simulink model "CLA_Sample"  (R2022b)
settings: Solver=FixedStepAuto  StartTime=0.0  StopTime=Inf  RelTol=1e-3  EnableMultiTasking=on
model workspace (MAT data in the model file):
  ADC_Gain = 1241.21212121
  DAC_Gain = 0.000805860805861
  Inductor_Current_Divider_Gain_Phase_A = 33.4
  Inductor_Current_Divider_Gain_Phase_B = 33.4
  Vbulk_Divider_Gain = 276.854928018
  Vin_Divider_Gain = 556.17352614
undefined symbols (not defined in the file or in its folder): GPTRIP1SEL, GPTRIP2SEL, SCI_A_Transmit, SCI_A_Transmit_Current_Suffix, SCI_A_Transmit_one_shot_Suffix, SCI_A_Transmit_Polarity_Suffix, SCI_A_Transmit_relay_Suffix, SCI_A_Transmit_Vbulk_Suffix, SCI_A_Transmit_Vin_rms_Suffix, SCI_A_Transmit_Vin_Suffix, SCI_A_Transmit_Vmid_Suffix, SCI_A_Transmit_Vp_Suffix, SCI_A_Transmit_Vpfc_Suffix, TZ1, TZ2
libraries: c280xlib x33, simulink x17, c2802xlib x15, c2000lib x1, c2806xlib x1
(part 1 of 5)
settings Model: ExtModeTrigDuration=8  Creator=natchammaimuthu  LastModifiedBy=hlaingwin
settings OptimizationCC: DefaultUnderspecifiedDataType=single  EnhancedBackFolding=on  PassReuseOutputArgsAs=Individual arguments  MaxStackSize=1024  OptimizeBlockOrder=speed  DifferentSizesBufferReuse=on  OptimizationCustomize=off  DenormalBehavior=FlushToZero  EfficientTunableParamExpr=on
settings DebuggingCC: MultiTaskDSMMsg=none  ParameterPrecisionLossMsg=none  ParameterTunabilityLossMsg=error
settings HardwareCC: ProdBitPerChar=16  ProdBitPerInt=16  ProdBitPerPointer=32  ProdBitPerSizeT=32  ProdBitPerPtrDiffT=32  ProdLargestAtomicInteger=Integer  ProdLargestAtomicFloat=None  ProdWordSize=16  ProdLongLongMode=on  ProdHWDeviceType=Texas Instruments->C2000
settings SFSimCC: MATLABDynamicMemAlloc=off
settings RTWCC: Description=Embedded Coder  SystemTargetFile=ert.tlc  HardwareBoard=TI Piccolo F2806x  TLCOptions=-aInlineSetEventsForThisBaseRateFcn=TLC_FALSE -aSuppressMultiTaskScheduler=TLC_FALSE -aRateBasedStepFcn=1  TemplateMakefile=ert_default_tmf  Toolchain=Texas Instruments Code Composer Studio (C2000)
settings CodeAppCC: ForceParamTrailComments=on  IgnoreCustomStorageClasses=off  OperatorAnnotations=on  SimulinkDataObjDesc=on  SFDataObjDesc=on  InsertBlockDesc=on
settings ERTTargetCC: CodeReplacementLibrary=TI C28x  ExtModeTransport=4  ExtModeStaticAlloc=on  ExtModeAutomaticAllocSize=off  ExtModeMexFile=ext_xcp  ExtModeIntrfLevel=Level2 - Open

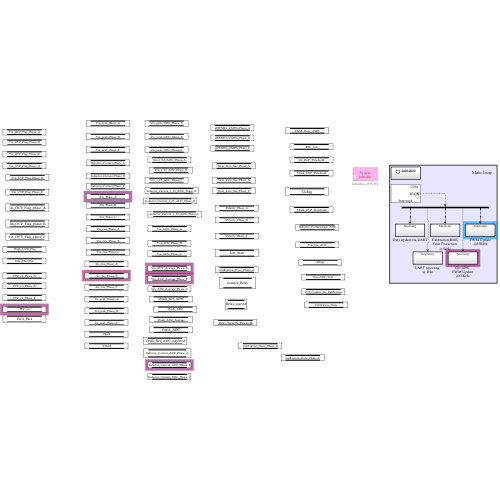
[thumbnail: Simulink's stored preview of the top-level diagram]
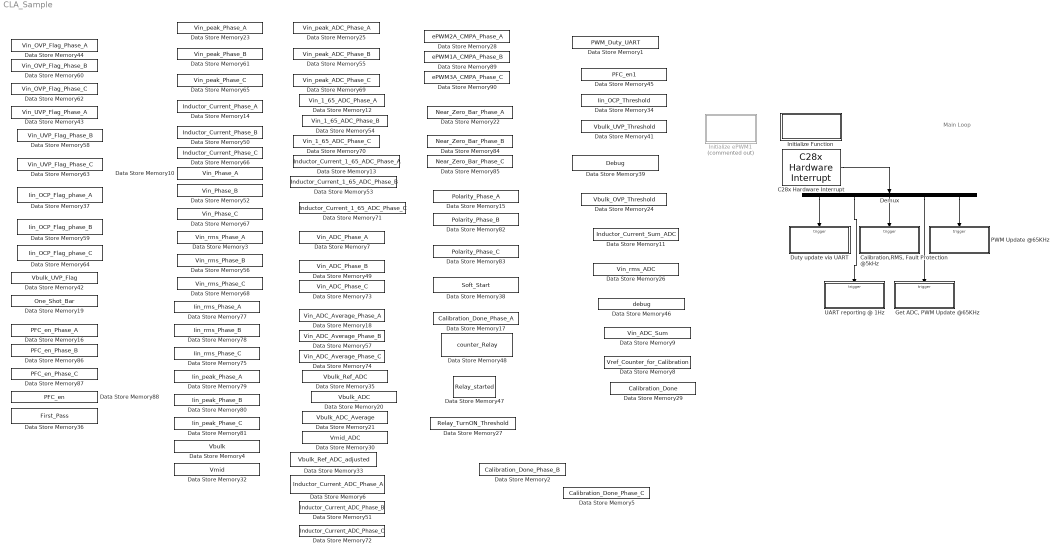
== system CLA_Sample ==
  note: Main Loop
  C28x Hardware Interrupt : c2000lib/Scheduling/C28x Hardware Interrupt  irqnumbers=[9 3 3 3 1]  pienumbers=[1 7 4 1 1]  irqpriorities=[10 9 8 7 6]  irqpreempts=[1 1 1 0 0]  showinput=off  dspchiptype=C280X
  "Calibration,RMS, Fault Protection @5kHz" : Subsystem  TreatAsAtomicUnit=on
  Data Store Memory1 : DataStoreMemory  DataStoreName=PWM_Duty_UART  WriteAfterWriteMsg=warning  InitialValue=5  ShowAdditionalParam=off  OutDataTypeStr=double
  Data Store Memory10 : DataStoreMemory  DataStoreName=Vin_Phase_A  WriteAfterWriteMsg=warning  ShowAdditionalParam=off  OutDataTypeStr=double
  Data Store Memory11 : DataStoreMemory  DataStoreName=Inductor_Current_Sum_ADC  WriteAfterWriteMsg=warning  ShowAdditionalParam=off  OutDataTypeStr=double
  Data Store Memory12 : DataStoreMemory  DataStoreName=Vin_1_65_ADC_Phase_A  WriteAfterWriteMsg=warning  ShowAdditionalParam=off  OutDataTypeStr=double
  Data Store Memory13 : DataStoreMemory  DataStoreName=Inductor_Current_1_65_ADC_Phase_A  WriteAfterWriteMsg=warning  ShowAdditionalParam=off  OutDataTypeStr=double
  Data Store Memory14 : DataStoreMemory  DataStoreName=Inductor_Current_Phase_A  WriteAfterWriteMsg=warning  ShowAdditionalParam=off  OutDataTypeStr=double
  Data Store Memory15 : DataStoreMemory  DataStoreName=Polarity_Phase_A  WriteAfterWriteMsg=warning  InitialValue=10  ShowAdditionalParam=off
  Data Store Memory16 : DataStoreMemory  DataStoreName=PFC_en_Phase_A  WriteAfterWriteMsg=warning  ShowAdditionalParam=off
  Data Store Memory17 : DataStoreMemory  DataStoreName=Calibration_Done_Phase_A  WriteAfterWriteMsg=warning  ShowAdditionalParam=off  OutDataTypeStr=double
  Data Store Memory18 : DataStoreMemory  DataStoreName=Vin_ADC_Average_Phase_A  WriteAfterWriteMsg=warning  ShowAdditionalParam=off
  Data Store Memory19 : DataStoreMemory  DataStoreName=One_Shot_Bar  WriteAfterWriteMsg=warning  InitialValue=1  ShowAdditionalParam=off  OutDataTypeStr=double
  Data Store Memory2 : DataStoreMemory  DataStoreName=Calibration_Done_Phase_B  WriteAfterWriteMsg=warning  ShowAdditionalParam=off  OutDataTypeStr=double
  Data Store Memory20 : DataStoreMemory  DataStoreName=Vbulk_ADC  WriteAfterWriteMsg=warning  ShowAdditionalParam=off
  Data Store Memory21 : DataStoreMemory  DataStoreName=Vbulk_ADC_Average  WriteAfterWriteMsg=warning  ShowAdditionalParam=off
  Data Store Memory22 : DataStoreMemory  DataStoreName=Near_Zero_Bar_Phase_A  WriteAfterWriteMsg=warning  InitialValue=10  ShowAdditionalParam=off
  Data Store Memory23 : DataStoreMemory  DataStoreName=Vin_peak_Phase_A  WriteAfterWriteMsg=warning  ShowAdditionalParam=off  OutDataTypeStr=double
  Data Store Memory24 : DataStoreMemory  DataStoreName=Vbulk_OVP_Threshold  WriteAfterWriteMsg=warning  InitialValue=100  ShowAdditionalParam=off
  Data Store Memory25 : DataStoreMemory  DataStoreName=Vin_peak_ADC_Phase_A  WriteAfterWriteMsg=warning  ShowAdditionalParam=off  OutDataTypeStr=double
  Data Store Memory26 : DataStoreMemory  DataStoreName=Vin_rms_ADC  WriteAfterWriteMsg=warning  InitialValue=10  ShowAdditionalParam=off
  Data Store Memory27 : DataStoreMemory  DataStoreName=Relay_TurnON_Threshold  WriteAfterWriteMsg=warning  InitialValue=10  ShowAdditionalParam=off
  Data Store Memory28 : DataStoreMemory  DataStoreName=ePWM2A_CMPA_Phase_A  WriteAfterWriteMsg=warning  ShowAdditionalParam=off
  Data Store Memory29 : DataStoreMemory  DataStoreName=Calibration_Done  WriteAfterWriteMsg=warning  ShowAdditionalParam=off  OutDataTypeStr=double
  Data Store Memory3 : DataStoreMemory  DataStoreName=Vin_rms_Phase_A  WriteAfterWriteMsg=warning  InitialValue=10  ShowAdditionalParam=off
  Data Store Memory30 : DataStoreMemory  DataStoreName=Vmid_ADC  WriteAfterWriteMsg=warning  InitialValue=10  ShowAdditionalParam=off  OutDataTypeStr=double
  Data Store Memory32 : DataStoreMemory  DataStoreName=Vmid  WriteAfterWriteMsg=warning  InitialValue=10  ShowAdditionalParam=off  OutDataTypeStr=double
  Data Store Memory33 : DataStoreMemory  DataStoreName=Vbulk_Ref_ADC_adjusted  WriteAfterWriteMsg=warning  InitialValue=10  ShowAdditionalParam=off  OutDataTypeStr=double
  Data Store Memory34 : DataStoreMemory  DataStoreName=Iin_OCP_Threshold  WriteAfterWriteMsg=warning  ShowAdditionalParam=off  OutDataTypeStr=double
  Data Store Memory35 : DataStoreMemory  DataStoreName=Vbulk_Ref_ADC  WriteAfterWriteMsg=warning  InitialValue=10  ShowAdditionalParam=off  OutDataTypeStr=double
  Data Store Memory36 : DataStoreMemory  DataStoreName=First_Pass  WriteAfterWriteMsg=warning  ShowAdditionalParam=off  OutDataTypeStr=double
  Data Store Memory37 : DataStoreMemory  DataStoreName=Iin_OCP_Flag_phase_A  WriteAfterWriteMsg=warning  InitialValue=1  ShowAdditionalParam=off  OutDataTypeStr=double
  Data Store Memory38 : DataStoreMemory  DataStoreName=Soft_Start  WriteAfterWriteMsg=warning  InitialValue=10  ShowAdditionalParam=off  OutDataTypeStr=double
  Data Store Memory39 : DataStoreMemory  DataStoreName=Debug  WriteAfterWriteMsg=warning  InitialValue=10  ShowAdditionalParam=off  OutDataTypeStr=double
  Data Store Memory4 : DataStoreMemory  DataStoreName=Vbulk  WriteAfterWriteMsg=warning  ShowAdditionalParam=off  OutDataTypeStr=double
  Data Store Memory41 : DataStoreMemory  DataStoreName=Vbulk_UVP_Threshold  WriteAfterWriteMsg=warning  InitialValue=-10  VectorParams1D=off  ShowAdditionalParam=off  OutDataTypeStr=double
  Data Store Memory42 : DataStoreMemory  DataStoreName=Vbulk_UVP_Flag  WriteAfterWriteMsg=warning  ShowAdditionalParam=off
  Data Store Memory43 : DataStoreMemory  DataStoreName=Vin_UVP_Flag_Phase_A  WriteAfterWriteMsg=warning  ShowAdditionalParam=off
  Data Store Memory44 : DataStoreMemory  DataStoreName=Vin_OVP_Flag_Phase_A  WriteAfterWriteMsg=warning  ShowAdditionalParam=off
  Data Store Memory45 : DataStoreMemory  DataStoreName=PFC_en1  WriteAfterWriteMsg=warning  ShowAdditionalParam=off
  Data Store Memory46 : DataStoreMemory  DataStoreName=debug  WriteAfterWriteMsg=warning  ShowAdditionalParam=off
  Data Store Memory47 : DataStoreMemory  DataStoreName=Relay_started  WriteAfterWriteMsg=warning  ShowAdditionalParam=off
  Data Store Memory48 : DataStoreMemory  DataStoreName=counter_Relay  WriteAfterWriteMsg=warning  ShowAdditionalParam=off
  Data Store Memory49 : DataStoreMemory  DataStoreName=Vin_ADC_Phase_B  WriteAfterWriteMsg=warning  ShowAdditionalParam=off
  Data Store Memory5 : DataStoreMemory  DataStoreName=Calibration_Done_Phase_C  WriteAfterWriteMsg=warning  ShowAdditionalParam=off  OutDataTypeStr=double
  Data Store Memory50 : DataStoreMemory  DataStoreName=Inductor_Current_Phase_B  WriteAfterWriteMsg=warning  ShowAdditionalParam=off  OutDataTypeStr=double
  Data Store Memory51 : DataStoreMemory  DataStoreName=Inductor_Current_ADC_Phase_B  WriteAfterWriteMsg=warning  ShowAdditionalParam=off  OutDataTypeStr=double
  Data Store Memory52 : DataStoreMemory  DataStoreName=Vin_Phase_B  WriteAfterWriteMsg=warning  ShowAdditionalParam=off  OutDataTypeStr=double
  Data Store Memory53 : DataStoreMemory  DataStoreName=Inductor_Current_1_65_ADC_Phase_B  WriteAfterWriteMsg=warning  ShowAdditionalParam=off  OutDataTypeStr=double
  Data Store Memory54 : DataStoreMemory  DataStoreName=Vin_1_65_ADC_Phase_B  WriteAfterWriteMsg=warning  ShowAdditionalParam=off  OutDataTypeStr=double
  Data Store Memory55 : DataStoreMemory  DataStoreName=Vin_peak_ADC_Phase_B  WriteAfterWriteMsg=warning  ShowAdditionalParam=off  OutDataTypeStr=double
  Data Store Memory56 : DataStoreMemory  DataStoreName=Vin_rms_Phase_B  WriteAfterWriteMsg=warning  InitialValue=10  ShowAdditionalParam=off
  Data Store Memory57 : DataStoreMemory  DataStoreName=Vin_ADC_Average_Phase_B  WriteAfterWriteMsg=warning  ShowAdditionalParam=off
  Data Store Memory58 : DataStoreMemory  DataStoreName=Vin_UVP_Flag_Phase_B  WriteAfterWriteMsg=warning  ShowAdditionalParam=off
  Data Store Memory59 : DataStoreMemory  DataStoreName=Iin_OCP_Flag_phase_B  WriteAfterWriteMsg=warning  InitialValue=1  ShowAdditionalParam=off  OutDataTypeStr=double
  Data Store Memory6 : DataStoreMemory  DataStoreName=Inductor_Current_ADC_Phase_A  WriteAfterWriteMsg=warning  ShowAdditionalParam=off  OutDataTypeStr=double
  Data Store Memory60 : DataStoreMemory  DataStoreName=Vin_OVP_Flag_Phase_B  WriteAfterWriteMsg=warning  ShowAdditionalParam=off
  Data Store Memory61 : DataStoreMemory  DataStoreName=Vin_peak_Phase_B  WriteAfterWriteMsg=warning  ShowAdditionalParam=off  OutDataTypeStr=double
  Data Store Memory62 : DataStoreMemory  DataStoreName=Vin_OVP_Flag_Phase_C  WriteAfterWriteMsg=warning  ShowAdditionalParam=off
  Data Store Memory63 : DataStoreMemory  DataStoreName=Vin_UVP_Flag_Phase_C  WriteAfterWriteMsg=warning  ShowAdditionalParam=off
  Data Store Memory64 : DataStoreMemory  DataStoreName=Iin_OCP_Flag_phase_C  WriteAfterWriteMsg=warning  InitialValue=1  ShowAdditionalParam=off  OutDataTypeStr=double
  Data Store Memory65 : DataStoreMemory  DataStoreName=Vin_peak_Phase_C  WriteAfterWriteMsg=warning  ShowAdditionalParam=off  OutDataTypeStr=double
  Data Store Memory66 : DataStoreMemory  DataStoreName=Inductor_Current_Phase_C  WriteAfterWriteMsg=warning  ShowAdditionalParam=off  OutDataTypeStr=double
  Data Store Memory67 : DataStoreMemory  DataStoreName=Vin_Phase_C  WriteAfterWriteMsg=warning  ShowAdditionalParam=off  OutDataTypeStr=double
  Data Store Memory68 : DataStoreMemory  DataStoreName=Vin_rms_Phase_C  WriteAfterWriteMsg=warning  InitialValue=10  ShowAdditionalParam=off
  Data Store Memory69 : DataStoreMemory  DataStoreName=Vin_peak_ADC_Phase_C  WriteAfterWriteMsg=warning  ShowAdditionalParam=off  OutDataTypeStr=double
  Data Store Memory7 : DataStoreMemory  DataStoreName=Vin_ADC_Phase_A  WriteAfterWriteMsg=warning  ShowAdditionalParam=off
  Data Store Memory70 : DataStoreMemory  DataStoreName=Vin_1_65_ADC_Phase_C  WriteAfterWriteMsg=warning  ShowAdditionalParam=off  OutDataTypeStr=double
  Data Store Memory71 : DataStoreMemory  DataStoreName=Inductor_Current_1_65_ADC_Phase_C  WriteAfterWriteMsg=warning  ShowAdditionalParam=off  OutDataTypeStr=double
  Data Store Memory72 : DataStoreMemory  DataStoreName=Inductor_Current_ADC_Phase_C  WriteAfterWriteMsg=warning  ShowAdditionalParam=off  OutDataTypeStr=double
  Data Store Memory73 : DataStoreMemory  DataStoreName=Vin_ADC_Phase_C  WriteAfterWriteMsg=warning  ShowAdditionalParam=off
  Data Store Memory74 : DataStoreMemory  DataStoreName=Vin_ADC_Average_Phase_C  WriteAfterWriteMsg=warning  ShowAdditionalParam=off
  Data Store Memory75 : DataStoreMemory  DataStoreName=Iin_rms_Phase_C  WriteAfterWriteMsg=warning  InitialValue=10  ShowAdditionalParam=off
  Data Store Memory77 : DataStoreMemory  DataStoreName=Iin_rms_Phase_A  WriteAfterWriteMsg=warning  InitialValue=10  ShowAdditionalParam=off
  Data Store Memory78 : DataStoreMemory  DataStoreName=Iin_rms_Phase_B  WriteAfterWriteMsg=warning  InitialValue=10  ShowAdditionalParam=off
  Data Store Memory79 : DataStoreMemory  DataStoreName=Iin_peak_Phase_A  WriteAfterWriteMsg=warning  ShowAdditionalParam=off  OutDataTypeStr=double
  Data Store Memory8 : DataStoreMemory  DataStoreName=Vref_Counter_for_Calibration  WriteAfterWriteMsg=warning  ShowAdditionalParam=off
  Data Store Memory80 : DataStoreMemory  DataStoreName=Iin_peak_Phase_B  WriteAfterWriteMsg=warning  ShowAdditionalParam=off  OutDataTypeStr=double
  Data Store Memory81 : DataStoreMemory  DataStoreName=Iin_peak_Phase_C  WriteAfterWriteMsg=warning  ShowAdditionalParam=off  OutDataTypeStr=double
  Data Store Memory82 : DataStoreMemory  DataStoreName=Polarity_Phase_B  WriteAfterWriteMsg=warning  InitialValue=10  ShowAdditionalParam=off
  Data Store Memory83 : DataStoreMemory  DataStoreName=Polarity_Phase_C  WriteAfterWriteMsg=warning  InitialValue=10  ShowAdditionalParam=off
  Data Store Memory84 : DataStoreMemory  DataStoreName=Near_Zero_Bar_Phase_B  WriteAfterWriteMsg=warning  InitialValue=10  ShowAdditionalParam=off
  Data Store Memory85 : DataStoreMemory  DataStoreName=Near_Zero_Bar_Phase_C  WriteAfterWriteMsg=warning  InitialValue=10  ShowAdditionalParam=off
  Data Store Memory86 : DataStoreMemory  DataStoreName=PFC_en_Phase_B  WriteAfterWriteMsg=warning  ShowAdditionalParam=off
  Data Store Memory87 : DataStoreMemory  DataStoreName=PFC_en_Phase_C  WriteAfterWriteMsg=warning  ShowAdditionalParam=off
  Data Store Memory88 : DataStoreMemory  DataStoreName=PFC_en  WriteAfterWriteMsg=warning  ShowAdditionalParam=off
  Data Store Memory89 : DataStoreMemory  DataStoreName=ePWM1A_CMPA_Phase_B  WriteAfterWriteMsg=warning  ShowAdditionalParam=off
  Data Store Memory9 : DataStoreMemory  DataStoreName=Vin_ADC_Sum  WriteAfterWriteMsg=warning  ShowAdditionalParam=off  OutDataTypeStr=double
  Data Store Memory90 : DataStoreMemory  DataStoreName=ePWM3A_CMPA_Phase_C  WriteAfterWriteMsg=warning  ShowAdditionalParam=off
  Demux : Demux  Outputs=5
  Duty update via UART : Subsystem  TreatAsAtomicUnit=on
  "Get ADC, PWM Update @65KHz" : Subsystem  TreatAsAtomicUnit=on
  Initialize Function : Subsystem  TreatAsAtomicUnit=on
  Initialize ePWM1 : Subsystem  Commented=on  mask(System Initialize){ShowInLibBrowser=0}
      mask prompts: ShowInLibBrowser "Simulink:masks:CustCodeMaskParam1_MP"
      settings: CopyFcn=cccopyfcn(gcb)  OpenFcn=ccopenfcn('System Initialize Function')
      mask Help: eval('feval(''rtwprivate'',''rtwhelpview'',''rtw_sys_initialize_block'')');
      mask Display: disp('System\nInitialize');
  PWM Update @65KHz : Subsystem  TreatAsAtomicUnit=on
  UART reporting @ 1Hz : Subsystem  TreatAsAtomicUnit=on
  wires:
  C28x Hardware Interrupt/1 -> Demux/1
  Demux/1 -> Duty update via UART/Trigger
  Demux/4 -> "Get ADC, PWM Update @65KHz"/Trigger
  Demux/5 -> PWM Update @65KHz/Trigger
  Demux/3 -> "Calibration,RMS, Fault Protection @5kHz"/Trigger
  Demux/2 -> UART reporting @ 1Hz/Trigger

== system CLA_Sample/Calibration,RMS, Fault Protection @5kHz ==
  function : TriggerPort  TriggerType=function-call  VariantControl=(inherit)
  Calibration : Subsystem  TreatAsAtomicUnit=on
  Fault checking : Subsystem  TreatAsAtomicUnit=on
  Function-Call Generator : simulink/Ports & Subsystems/Function-Call Generator  sample_time=-1  numberOfIterations=1  DisallowWideOutput=off
  Function-Call Split : FunctionCallSplit  IconShape=distinctive  NumOutputPorts=6  OutputPortLayout=default
  Polarity & Near Zero check : Subsystem  Commented=on  TreatAsAtomicUnit=on
  Relay control : Subsystem  TreatAsAtomicUnit=on
  Soft Start : Subsystem  TreatAsAtomicUnit=on
  Voltage RMS/Averag Calculation : Subsystem  TreatAsAtomicUnit=on
  wires:
  Function-Call Generator/1 -> Function-Call Split/1
  Function-Call Split/1 -> Calibration/Trigger
  Function-Call Split/2 -> Voltage RMS/Averag Calculation/Trigger
  Function-Call Split/3 -> Fault checking/Trigger
  Function-Call Split/4 -> Polarity & Near Zero check/Trigger
  Function-Call Split/5 -> Relay control/Trigger
  Function-Call Split/6 -> Soft Start/Trigger

== system CLA_Sample/Duty update via UART ==
  function : TriggerPort  TriggerType=function-call  VariantControl=(inherit)
  Data Store Write1 : DataStoreWrite  DataStoreName=PWM_Duty_UART  IndexOptions=Index vector (dialog)  Indices=1  OutputSizes=1
  Function Caller : FunctionCaller  FunctionPrototype=y = SCI_Receive()  InputArgumentSpecifications=<Enter example>  OutputArgumentSpecifications=<Enter example>
  Simulink Function : Subsystem  TreatAsAtomicUnit=on
  wires:
  Function Caller/1 -> Data Store Write1/1

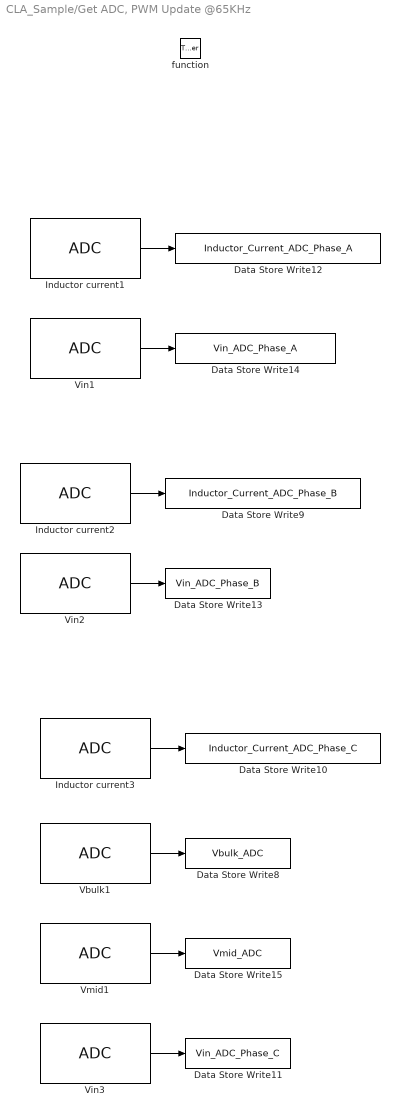
== system CLA_Sample/Get ADC, PWM Update @65KHz ==
  function : TriggerPort  TriggerType=function-call  VariantControl=(inherit)
  Data Store Write10 : DataStoreWrite  DataStoreName=Inductor_Current_ADC_Phase_C  IndexOptions=Index vector (dialog)  Indices=1  OutputSizes=1
  Data Store Write11 : DataStoreWrite  DataStoreName=Vin_ADC_Phase_C  IndexOptions=Index vector (dialog)  Indices=1  OutputSizes=1
  Data Store Write12 : DataStoreWrite  DataStoreName=Inductor_Current_ADC_Phase_A  IndexOptions=Index vector (dialog)  Indices=1  OutputSizes=1
  Data Store Write13 : DataStoreWrite  DataStoreName=Vin_ADC_Phase_B  IndexOptions=Index vector (dialog)  Indices=1  OutputSizes=1
  Data Store Write14 : DataStoreWrite  DataStoreName=Vin_ADC_Phase_A  IndexOptions=Index vector (dialog)  Indices=1  OutputSizes=1
  Data Store Write15 : DataStoreWrite  DataStoreName=Vmid_ADC  IndexOptions=Index vector (dialog)  Indices=1  OutputSizes=1
  Data Store Write8 : DataStoreWrite  DataStoreName=Vbulk_ADC  IndexOptions=Index vector (dialog)  Indices=1  OutputSizes=1
  Data Store Write9 : DataStoreWrite  DataStoreName=Inductor_Current_ADC_Phase_B  IndexOptions=Index vector (dialog)  Indices=1  OutputSizes=1
  Inductor current1 : c2802xlib/ADC  blkParamProc=C2000  ADCModule=1  samplingMode=Single sample mode  ADCResolution=12-bit (Single-ended input)  useSOC1=SOC4  useSOC2=SOC0_SOC1  SOCAcquisitionWindow=10  SOCTriggerSource=ePWM1_ADCSOCA  SOCInterruptTrigger=No ADCINT  Ts=-1  dType=double  postInterrupt=off  interruptSel=ADCINT1  ADCINTContinuous=off  endma=off  chdma=1  conv1=ADCINA2  conv2=ADCINA0 and ADCINB0  conv1_Type4=ADCIN0  conv2_Type4=ADCIN0 and ADCIN1
      settings: LibrarySourceBlock=c2806xlib/ADC
  Inductor current2 : c2802xlib/ADC  blkParamProc=C2000  ADCModule=1  samplingMode=Single sample mode  ADCResolution=12-bit (Single-ended input)  useSOC1=SOC0  useSOC2=SOC0_SOC1  SOCAcquisitionWindow=10  SOCTriggerSource=ePWM1_ADCSOCA  SOCInterruptTrigger=No ADCINT  Ts=-1  dType=double  postInterrupt=off  interruptSel=ADCINT1  ADCINTContinuous=off  endma=off  chdma=1  conv1=ADCINA1  conv2=ADCINA0 and ADCINB0  conv1_Type4=ADCIN0  conv2_Type4=ADCIN0 and ADCIN1
      settings: LibrarySourceBlock=c2806xlib/ADC
  Inductor current3 : c2802xlib/ADC  blkParamProc=C2000  ADCModule=1  samplingMode=Single sample mode  ADCResolution=12-bit (Single-ended input)  useSOC1=SOC6  useSOC2=SOC0_SOC1  SOCAcquisitionWindow=10  SOCTriggerSource=ePWM1_ADCSOCA  SOCInterruptTrigger=No ADCINT  Ts=-1  dType=double  postInterrupt=off  interruptSel=ADCINT1  ADCINTContinuous=off  endma=off  chdma=1  conv1=ADCINA0  conv2=ADCINA0 and ADCINB0  conv1_Type4=ADCIN0  conv2_Type4=ADCIN0 and ADCIN1
      settings: LibrarySourceBlock=c2806xlib/ADC
  Vbulk1 : c2802xlib/ADC  blkParamProc=C2000  ADCModule=1  samplingMode=Single sample mode  ADCResolution=12-bit (Single-ended input)  useSOC1=SOC3  useSOC2=SOC0_SOC1  SOCAcquisitionWindow=10  SOCTriggerSource=ePWM1_ADCSOCA  SOCInterruptTrigger=No ADCINT  Ts=-1  dType=double  postInterrupt=off  interruptSel=ADCINT1  ADCINTContinuous=off  endma=off  chdma=1  conv1=ADCINA3  conv2=ADCINA0 and ADCINB0  conv1_Type4=ADCIN0  conv2_Type4=ADCIN0 and ADCIN1
      settings: LibrarySourceBlock=c2806xlib/ADC
  Vin1 : c2802xlib/ADC  blkParamProc=C2000  ADCModule=1  samplingMode=Single sample mode  ADCResolution=12-bit (Single-ended input)  useSOC1=SOC5  useSOC2=SOC0_SOC1  SOCAcquisitionWindow=10  SOCTriggerSource=ePWM1_ADCSOCA  SOCInterruptTrigger=No ADCINT  Ts=-1  dType=double  postInterrupt=off  interruptSel=ADCINT1  ADCINTContinuous=off  endma=off  chdma=1  conv1=ADCINB2  conv2=ADCINA0 and ADCINB0  conv1_Type4=ADCIN0  conv2_Type4=ADCIN0 and ADCIN1
      settings: LibrarySourceBlock=c2806xlib/ADC
  Vin2 : c2802xlib/ADC  blkParamProc=C2000  ADCModule=1  samplingMode=Single sample mode  ADCResolution=12-bit (Single-ended input)  useSOC1=SOC1  useSOC2=SOC0_SOC1  SOCAcquisitionWindow=10  SOCTriggerSource=ePWM1_ADCSOCA  SOCInterruptTrigger=No ADCINT  Ts=-1  dType=double  postInterrupt=off  interruptSel=ADCINT1  ADCINTContinuous=off  endma=off  chdma=1  conv1=ADCINB1  conv2=ADCINA0 and ADCINB0  conv1_Type4=ADCIN0  conv2_Type4=ADCIN0 and ADCIN1
      settings: LibrarySourceBlock=c2806xlib/ADC
  Vin3 : c2802xlib/ADC  blkParamProc=C2000  ADCModule=1  samplingMode=Single sample mode  ADCResolution=12-bit (Single-ended input)  useSOC1=SOC7  useSOC2=SOC0_SOC1  SOCAcquisitionWindow=10  SOCTriggerSource=ePWM1_ADCSOCA  SOCInterruptTrigger=No ADCINT  Ts=-1  dType=double  postInterrupt=on  interruptSel=ADCINT1  ADCINTContinuous=on  endma=off  chdma=1  conv1=ADCINB0  conv2=ADCINA0 and ADCINB0  conv1_Type4=ADCIN0  conv2_Type4=ADCIN0 and ADCIN1
      settings: LibrarySourceBlock=c2806xlib/ADC
  Vmid1 : c2802xlib/ADC  blkParamProc=C2000  ADCModule=1  samplingMode=Single sample mode  ADCResolution=12-bit (Single-ended input)  useSOC1=SOC2  useSOC2=SOC0_SOC1  SOCAcquisitionWindow=10  SOCTriggerSource=ePWM1_ADCSOCA  SOCInterruptTrigger=No ADCINT  Ts=-1  dType=double  postInterrupt=off  interruptSel=ADCINT1  ADCINTContinuous=on  endma=off  chdma=1  conv1=ADCINA4  conv2=ADCINA0 and ADCINB0  conv1_Type4=ADCIN0  conv2_Type4=ADCIN0 and ADCIN1
      settings: LibrarySourceBlock=c2806xlib/ADC
  wires:
  Inductor current1/1 -> Data Store Write12/1
  Vin3/1 -> Data Store Write11/1
  Vin2/1 -> Data Store Write13/1
  Vbulk1/1 -> Data Store Write8/1
  Vmid1/1 -> Data Store Write15/1
  Inductor current2/1 -> Data Store Write9/1
  Vin1/1 -> Data Store Write14/1
  Inductor current3/1 -> Data Store Write10/1

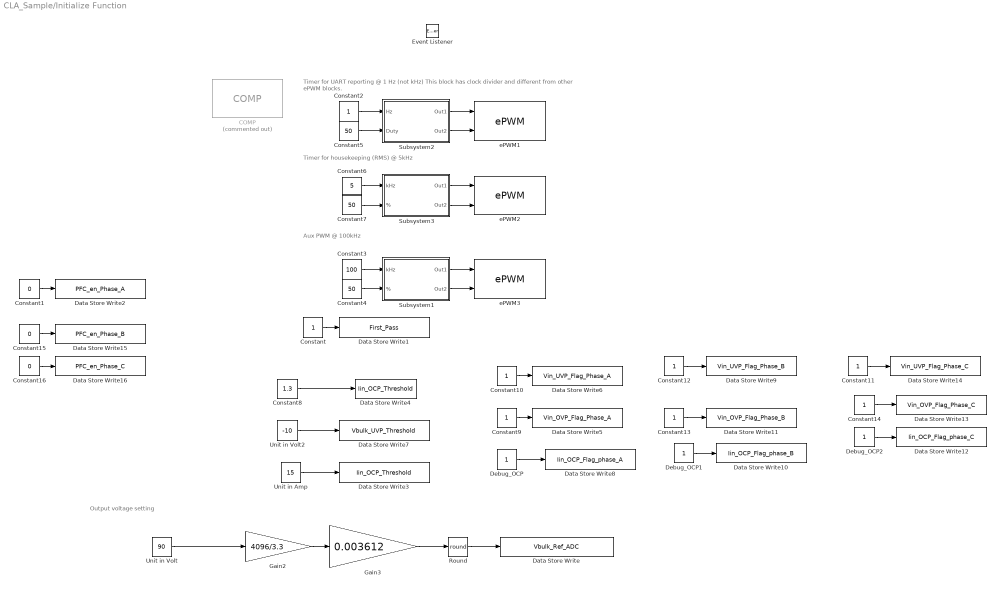
== system CLA_Sample/Initialize Function ==
  note: Aux PWM @ 100kHz
  note: Timer for UART reporting @ 1 Hz (not kHz)
      | This block has clock divider and different from other ePWM blocks.
  note: Timer for housekeeping (RMS) @ 5kHz
  note: Output voltage setting
  COMP : c2802xlib/COMP  Commented=on  comparatorModule=Comparator 1  comparatorGPIO1=[]  comparatorGPIO2=0  comparatorSource=Internal DAC  DACOutputValue=1023  inverterCircuit=off  synchronizationSelect=Asynchronous  qualificationPeriod=Passed through  Ts=-1
      settings: LibrarySourceBlock=c2806xlib/COMP
  Constant{,2,9..14} (8 alike) : Constant
  Constant1 : Constant  Value=0
  Constant15 : Constant  Value=0
  Constant16 : Constant  Value=0
  Constant3 : Constant  Value=100
  Constant4 : Constant  Value=50
  Constant5 : Constant  Value=50
  Constant6 : Constant  Value=5
  Constant7 : Constant  Value=50
  Constant8 : Constant  Value=1.3
  Data Store Write : DataStoreWrite  DataStoreName=Vbulk_Ref_ADC  IndexOptions=Index vector (dialog)  Indices=1  OutputSizes=1
  Data Store Write1 : DataStoreWrite  DataStoreName=First_Pass  IndexOptions=Index vector (dialog)  Indices=1  OutputSizes=1
  Data Store Write10 : DataStoreWrite  DataStoreName=Iin_OCP_Flag_phase_B  IndexOptions=Index vector (dialog)  Indices=1  OutputSizes=1
  Data Store Write11 : DataStoreWrite  DataStoreName=Vin_OVP_Flag_Phase_B  IndexOptions=Index vector (dialog)  Indices=1  OutputSizes=1
  Data Store Write12 : DataStoreWrite  DataStoreName=Iin_OCP_Flag_phase_C  IndexOptions=Index vector (dialog)  Indices=1  OutputSizes=1
  Data Store Write13 : DataStoreWrite  DataStoreName=Vin_OVP_Flag_Phase_C  IndexOptions=Index vector (dialog)  Indices=1  OutputSizes=1
  Data Store Write14 : DataStoreWrite  DataStoreName=Vin_UVP_Flag_Phase_C  IndexOptions=Index vector (dialog)  Indices=1  OutputSizes=1
  Data Store Write15 : DataStoreWrite  DataStoreName=PFC_en_Phase_B  IndexOptions=Index vector (dialog)  Indices=1  OutputSizes=1
  Data Store Write16 : DataStoreWrite  DataStoreName=PFC_en_Phase_C  IndexOptions=Index vector (dialog)  Indices=1  OutputSizes=1
  Data Store Write2 : DataStoreWrite  DataStoreName=PFC_en_Phase_A  IndexOptions=Index vector (dialog)  Indices=1  OutputSizes=1
  Data Store Write3 : DataStoreWrite  DataStoreName=Iin_OCP_Threshold  IndexOptions=Index vector (dialog)  Indices=1  OutputSizes=1
  Data Store Write4 : DataStoreWrite  DataStoreName=Iin_OCP_Threshold  IndexOptions=Index vector (dialog)  Indices=1  OutputSizes=1
  Data Store Write5 : DataStoreWrite  DataStoreName=Vin_OVP_Flag_Phase_A  IndexOptions=Index vector (dialog)  Indices=1  OutputSizes=1
  Data Store Write6 : DataStoreWrite  DataStoreName=Vin_UVP_Flag_Phase_A  IndexOptions=Index vector (dialog)  Indices=1  OutputSizes=1
  Data Store Write7 : DataStoreWrite  DataStoreName=Vbulk_UVP_Threshold  IndexOptions=Index vector (dialog)  Indices=1  OutputSizes=1
  Data Store Write8 : DataStoreWrite  DataStoreName=Iin_OCP_Flag_phase_A  IndexOptions=Index vector (dialog)  Indices=1  OutputSizes=1
  Data Store Write9 : DataStoreWrite  DataStoreName=Vin_UVP_Flag_Phase_B  IndexOptions=Index vector (dialog)  Indices=1  OutputSizes=1
  Debug_OCP : Constant
  Debug_OCP1 : Constant
  Debug_OCP2 : Constant
  Event Listener : EventListener  DisableCoverage=on  EventName=reset
  Gain2 : Gain  Gain=4096/3.3
  Gain3 : Gain  Gain=0.003612  OutDataTypeStr=double
  Round : Rounding  Operator=round
  Subsystem1 : Subsystem
  Subsystem2 : Subsystem
  Subsystem3 : Subsystem
  Unit in Amp : Constant  Value=15
  Unit in Volt : Constant  Value=90
  Unit in Volt2 : Constant  Value=-10
  ePWM1 : c2802xlib/ePWM  PwmType=C2000  useModule=ePWM7  ePWMxLINKTBPRD=Not Linked  periodUnits=Clock cycles  timerSource=Input port  timerPeriod_clk=50224  timerPeriod_sec=0.0001  tbshadow=Counter equals to zero  countingMode=Up  phaseActiveEnable=Disable  phaseDirection=Count down after sync  phaseActive=0  synchronizationEnable=off  dcaevt1Sync=off  dcbevt1Sync=off  synchronizationOption=Disable  dcbevt1SyncOut=off  dcaevt1SyncOut=off  cmpdSyncOut=off  cmpcSyncOut=off  cmpbSyncOut=off  zeroSyncOut=off  swfSyncOut=off  perSynchronizationOption=Counter equals to period (CTR=PRD)  clockPrescale=128  HSclockPrescale=14  enswap=off  ePWMxAStatus=on  ePWMxAactionLogic1=Clear  ePWMxAactionLogic2=Do nothing  ePWMxAactionLogic3=Set  ePWMxAactionLogic4=Set  ePWMxAactionLogic5=Do nothing  ePWMxAactionLogic6=Do nothing  ePWMxACSFenable=off  ePWMxACSFvalue=Forcing disable  ePWMxASFreload=Zero  ePWMxBStatus=off  ePWMxBactionLogic1=Set  ePWMxBactionLogic2=Do nothing  ePWMxBactionLogic3=Clear  ePWMxBactionLogic4=Do nothing  ePWMxBactionLogic5=Do nothing  ePWMxBactionLogic6=Set  ePWMxBCSFenable=off  ePWMxBCSFvalue=Forcing disable  ePWMxBSFreload=Zero  ePWNxBOutWay=off  ePWMxLINKCMPA=Not Linked  CMPAUnits=Clock cycles  CMPASource=Input port  CMPAValue_per=50  CMPAValue_clk=32000  enCMPAshadow=Counter equals to zero (CTR=Zero)  ePWMxLINKCMPB=Not Linked  CMPBUnits=Clock cycles  CMPBSource=Specify via dialog  CMPBValue_per=50  CMPBValue_clk=32000  enCMPBshadow=Counter equals to zero (CTR=Zero)  ePWMxLINKCMPC=Not Linked  CMPCUnits=Clock cycles  CMPCSource=Specify via dialog  CMPCValue_per=50  CMPCValue_clk=32000  enCMPCshadow=Counter equals to zero (CTR=Zero)  ePWMxLINKCMPD=Not Linked  CMPDUnits=Clock cycles  CMPDSource=Specify via dialog  CMPDValue_per=50  CMPDValue_clk=32000  enCMPDshadow=Counter equals to zero (CTR=Zero)  enableDBePWMxA=off  enableDBePWMxB=off  enhalfcycle=off  DBpolarity=Active high (AH)  DBedgeDelay=Positive  DBSource_ePWMxA=ePWMxA  DBSource_ePWMxB=ePWMxA  DBPeriodUnits=Clock cycles  DBperiodSource=Specify via dialog  REDperiod=0  FEDperiod=0  REDperiod_sec=0  FEDperiod_sec=0  LoadModeDBRED=Immediate without using shadow  LoadModeDBFED=Immediate without using shadow  adcstartModuleA=off  adcrequestEventA=First event  adcstartEventA=Counter equals to zero (CTR=Zero)  adcstartEventA_type2=Digital Compare Module A Event 1 start of conversion (DCAEVT1.soc)  adcstartModuleB=off  adcrequestEventB=First event  adcstartEventB=Counter equals to zero (CTR=Zero)  adcstartEventB_type2=Counter equals to zero (CTR=Zero)  intEn=on  intPrd=First event  intSel=Counter equals to zero (CTR=Zero)  intSel_type2=Counter equals to zero (CTR=Zero)  hrpe=off  enHRPWM=off  HRPWM_LoadMode=Counter equals to period (CTR=PRD)  HRPWM_CTLMode=Duty or Period control mode  HRPWM_EDGMode=Both edge  hrpeb=off  enHRPWMB=off  HRPWM_LoadModeB=Counter equals to zero (CTR=ZERO)  HRPWM_CTLModeB=Duty or Period control mode  HRPWM_EDGModeB=Both edge  enHRDBRED=off  enHRDBFED=off  enSFO=on  enautoconv=on  chopperEnable=off  chopperFrequency=1  chopperFirstwidth=1  chopperDuty=12.5%  tripZonesource=Specify via dialog  tzselOSHT1=off  tzselOSHT2=off  tzselOSHT3=off  tzselOSHDCAEV1=off  tzselOSHDCBEV1=off  tzselCBC1=off  tzselCBC2=off  tzselCBC3=off  tzselCBCDCAEV2=off  tzselCBCDCBEV2=off  tzselOSHT4=off  tzselOSHT5=off  tzselOSHT6=off  tzselCBC4=off  tzselCBC5=off  tzselCBC6=off  enTzOstIntr=off  enTzCbcIntr=off  enTzDCAEVT1Intr=off  enTzDCAEVT2Intr=off  enTzDCBEVT1Intr=off  enTzDCBEVT2Intr=off  ePWMxAforced=No action  ePWMxBforced=No action  DCAEVT1forced=No action  DCBEVT1forced=No action  DCAEVT2forced=No action  DCBEVT2forced=No action  dcah=Trip Zone 1 input (TZ1)  dcal=Trip Zone 1 input (TZ1)  dcbh=Trip Zone 1 input (TZ1)  dcbl=Trip Zone 1 input (TZ1)  dcah_type2=GPTRIP1SEL/(TZ1)  dcal_type2=GPTRIP2SEL/(TZ2)  dcbh_type2=GPTRIP1SEL/(TZ1)  dcbl_type2=GPTRIP2SEL/(TZ2)  gendcaevt1=Event disabled  gendcaevt2=Event disabled  gendcbevt1=Event disabled  gendcbevt2=Event disabled  dcaevt1src=DCAEVT1 with sync  dcaevt2src=DCAEVT2 with sync  dcbevt1src=DCBEVT1 with sync  dcbevt2src=DCBEVT2 with sync  pulsesel=Counter equals to zero (CTR=Zero)  blankinv=off  blankoffset=0  blankwidth=0  evsrcsel=Filtered version of DCAEVT1 (DCAEVT1FILT)  encape=off
      settings: LibrarySourceBlock=c2806xlib/ePWM
  ePWM2 : c2802xlib/ePWM  PwmType=C2000  useModule=ePWM4  ePWMxLINKTBPRD=Not Linked  periodUnits=Clock cycles  timerSource=Input port  timerPeriod_clk=64000  timerPeriod_sec=0.0001  tbshadow=Counter equals to zero  countingMode=Up  phaseActiveEnable=Disable  phaseDirection=Count down after sync  phaseActive=0  synchronizationEnable=off  dcaevt1Sync=off  dcbevt1Sync=off  synchronizationOption=Disable  dcbevt1SyncOut=off  dcaevt1SyncOut=off  cmpdSyncOut=off  cmpcSyncOut=off  cmpbSyncOut=off  zeroSyncOut=off  swfSyncOut=off  perSynchronizationOption=Counter equals to period (CTR=PRD)  clockPrescale=1  HSclockPrescale=1  enswap=off  ePWMxAStatus=on  ePWMxAactionLogic1=Clear  ePWMxAactionLogic2=Do nothing  ePWMxAactionLogic3=Set  ePWMxAactionLogic4=Set  ePWMxAactionLogic5=Do nothing  ePWMxAactionLogic6=Do nothing  ePWMxACSFenable=off  ePWMxACSFvalue=Forcing disable  ePWMxASFreload=Zero  ePWMxBStatus=off  ePWMxBactionLogic1=Set  ePWMxBactionLogic2=Do nothing  ePWMxBactionLogic3=Clear  ePWMxBactionLogic4=Do nothing  ePWMxBactionLogic5=Do nothing  ePWMxBactionLogic6=Set  ePWMxBCSFenable=off  ePWMxBCSFvalue=Forcing disable  ePWMxBSFreload=Zero  ePWNxBOutWay=off  ePWMxLINKCMPA=Not Linked  CMPAUnits=Clock cycles  CMPASource=Input port  CMPAValue_per=50  CMPAValue_clk=32000  enCMPAshadow=Counter equals to zero (CTR=Zero)  ePWMxLINKCMPB=Not Linked  CMPBUnits=Clock cycles  CMPBSource=Specify via dialog  CMPBValue_per=50  CMPBValue_clk=32000  enCMPBshadow=Counter equals to zero (CTR=Zero)  ePWMxLINKCMPC=Not Linked  CMPCUnits=Clock cycles  CMPCSource=Specify via dialog  CMPCValue_per=50  CMPCValue_clk=32000  enCMPCshadow=Counter equals to zero (CTR=Zero)  ePWMxLINKCMPD=Not Linked  CMPDUnits=Clock cycles  CMPDSource=Specify via dialog  CMPDValue_per=50  CMPDValue_clk=32000  enCMPDshadow=Counter equals to zero (CTR=Zero)  enableDBePWMxA=off  enableDBePWMxB=off  enhalfcycle=off  DBpolarity=Active high (AH)  DBedgeDelay=Positive  DBSource_ePWMxA=ePWMxA  DBSource_ePWMxB=ePWMxA  DBPeriodUnits=Clock cycles  DBperiodSource=Specify via dialog  REDperiod=0  FEDperiod=0  REDperiod_sec=0  FEDperiod_sec=0  LoadModeDBRED=Immediate without using shadow  LoadModeDBFED=Immediate without using shadow  adcstartModuleA=off  adcrequestEventA=First event  adcstartEventA=Counter equals to zero (CTR=Zero)  adcstartEventA_type2=Digital Compare Module A Event 1 start of conversion (DCAEVT1.soc)  adcstartModuleB=off  adcrequestEventB=First event  adcstartEventB=Counter equals to zero (CTR=Zero)  adcstartEventB_type2=Counter equals to zero (CTR=Zero)  intEn=on  intPrd=First event  intSel=Counter equals to zero (CTR=Zero)  intSel_type2=Counter equals to zero (CTR=Zero)  hrpe=off  enHRPWM=off  HRPWM_LoadMode=Counter equals to period (CTR=PRD)  HRPWM_CTLMode=Duty or Period control mode  HRPWM_EDGMode=Both edge  hrpeb=off  enHRPWMB=off  HRPWM_LoadModeB=Counter equals to zero (CTR=ZERO)  HRPWM_CTLModeB=Duty or Period control mode  HRPWM_EDGModeB=Both edge  enHRDBRED=off  enHRDBFED=off  enSFO=on  enautoconv=on  chopperEnable=off  chopperFrequency=1  chopperFirstwidth=1  chopperDuty=12.5%  tripZonesource=Specify via dialog  tzselOSHT1=off  tzselOSHT2=off  tzselOSHT3=off  tzselOSHDCAEV1=off  tzselOSHDCBEV1=off  tzselCBC1=off  tzselCBC2=off  tzselCBC3=off  tzselCBCDCAEV2=off  tzselCBCDCBEV2=off  tzselOSHT4=off  tzselOSHT5=off  tzselOSHT6=off  tzselCBC4=off  tzselCBC5=off  tzselCBC6=off  enTzOstIntr=off  enTzCbcIntr=off  enTzDCAEVT1Intr=off  enTzDCAEVT2Intr=off  enTzDCBEVT1Intr=off  enTzDCBEVT2Intr=off  ePWMxAforced=No action  ePWMxBforced=No action  DCAEVT1forced=No action  DCBEVT1forced=No action  DCAEVT2forced=No action  DCBEVT2forced=No action  dcah=Trip Zone 1 input (TZ1)  dcal=Trip Zone 1 input (TZ1)  dcbh=Trip Zone 1 input (TZ1)  dcbl=Trip Zone 1 input (TZ1)  dcah_type2=GPTRIP1SEL/(TZ1)  dcal_type2=GPTRIP2SEL/(TZ2)  dcbh_type2=GPTRIP1SEL/(TZ1)  dcbl_type2=GPTRIP2SEL/(TZ2)  gendcaevt1=Event disabled  gendcaevt2=Event disabled  gendcbevt1=Event disabled  gendcbevt2=Event disabled  dcaevt1src=DCAEVT1 with sync  dcaevt2src=DCAEVT2 with sync  dcbevt1src=DCBEVT1 with sync  dcbevt2src=DCBEVT2 with sync  pulsesel=Counter equals to zero (CTR=Zero)  blankinv=off  blankoffset=0  blankwidth=0  evsrcsel=Filtered version of DCAEVT1 (DCAEVT1FILT)  encape=off
      settings: LibrarySourceBlock=c2806xlib/ePWM
  ePWM3 : c2802xlib/ePWM  PwmType=C2000  useModule=ePWM8  ePWMxLINKTBPRD=Not Linked  periodUnits=Clock cycles  timerSource=Input port  timerPeriod_clk=64000  timerPeriod_sec=0.0001  tbshadow=Counter equals to zero  countingMode=Up  phaseActiveEnable=Disable  phaseDirection=Count down after sync  phaseActive=0  synchronizationEnable=off  dcaevt1Sync=off  dcbevt1Sync=off  synchronizationOption=Disable  dcbevt1SyncOut=off  dcaevt1SyncOut=off  cmpdSyncOut=off  cmpcSyncOut=off  cmpbSyncOut=off  zeroSyncOut=off  swfSyncOut=off  perSynchronizationOption=Counter equals to period (CTR=PRD)  clockPrescale=1  HSclockPrescale=1  enswap=off  ePWMxAStatus=on  ePWMxAactionLogic1=Clear  ePWMxAactionLogic2=Do nothing  ePWMxAactionLogic3=Set  ePWMxAactionLogic4=Set  ePWMxAactionLogic5=Do nothing  ePWMxAactionLogic6=Do nothing  ePWMxACSFenable=off  ePWMxACSFvalue=Forcing disable  ePWMxASFreload=Zero  ePWMxBStatus=on  ePWMxBactionLogic1=Set  ePWMxBactionLogic2=Do nothing  ePWMxBactionLogic3=Clear  ePWMxBactionLogic4=Do nothing  ePWMxBactionLogic5=Do nothing  ePWMxBactionLogic6=Set  ePWMxBCSFenable=off  ePWMxBCSFvalue=Forcing disable  ePWMxBSFreload=Zero  ePWNxBOutWay=off  ePWMxLINKCMPA=Not Linked  CMPAUnits=Clock cycles  CMPASource=Input port  CMPAValue_per=50  CMPAValue_clk=32000  enCMPAshadow=Counter equals to zero (CTR=Zero)  ePWMxLINKCMPB=Not Linked  CMPBUnits=Clock cycles  CMPBSource=Specify via dialog  CMPBValue_per=50  CMPBValue_clk=32000  enCMPBshadow=Counter equals to zero (CTR=Zero)  ePWMxLINKCMPC=Not Linked  CMPCUnits=Clock cycles  CMPCSource=Specify via dialog  CMPCValue_per=50  CMPCValue_clk=32000  enCMPCshadow=Counter equals to zero (CTR=Zero)  ePWMxLINKCMPD=Not Linked  CMPDUnits=Clock cycles  CMPDSource=Specify via dialog  CMPDValue_per=50  CMPDValue_clk=32000  enCMPDshadow=Counter equals to zero (CTR=Zero)  enableDBePWMxA=off  enableDBePWMxB=off  enhalfcycle=off  DBpolarity=Active high (AH)  DBedgeDelay=Positive  DBSource_ePWMxA=ePWMxA  DBSource_ePWMxB=ePWMxA  DBPeriodUnits=Clock cycles  DBperiodSource=Specify via dialog  REDperiod=0  FEDperiod=0  REDperiod_sec=0  FEDperiod_sec=0  LoadModeDBRED=Immediate without using shadow  LoadModeDBFED=Immediate without using shadow  adcstartModuleA=off  adcrequestEventA=First event  adcstartEventA=Counter equals to zero (CTR=Zero)  adcstartEventA_type2=Digital Compare Module A Event 1 start of conversion (DCAEVT1.soc)  adcstartModuleB=off  adcrequestEventB=First event  adcstartEventB=Counter equals to zero (CTR=Zero)  adcstartEventB_type2=Counter equals to zero (CTR=Zero)  intEn=off  intPrd=First event  intSel=Counter equals to zero (CTR=Zero)  intSel_type2=Counter equals to zero (CTR=Zero)  hrpe=off  enHRPWM=off  HRPWM_LoadMode=Counter equals to period (CTR=PRD)  HRPWM_CTLMode=Duty or Period control mode  HRPWM_EDGMode=Both edge  hrpeb=off  enHRPWMB=off  HRPWM_LoadModeB=Counter equals to zero (CTR=ZERO)  HRPWM_CTLModeB=Duty or Period control mode  HRPWM_EDGModeB=Both edge  enHRDBRED=off  enHRDBFED=off  enSFO=on  enautoconv=on  chopperEnable=off  chopperFrequency=1  chopperFirstwidth=1  chopperDuty=12.5%  tripZonesource=Specify via dialog  tzselOSHT1=off  tzselOSHT2=off  tzselOSHT3=off  tzselOSHDCAEV1=off  tzselOSHDCBEV1=off  tzselCBC1=off  tzselCBC2=off  tzselCBC3=off  tzselCBCDCAEV2=off  tzselCBCDCBEV2=off  tzselOSHT4=off  tzselOSHT5=off  tzselOSHT6=off  tzselCBC4=off  tzselCBC5=off  tzselCBC6=off  enTzOstIntr=off  enTzCbcIntr=off  enTzDCAEVT1Intr=off  enTzDCAEVT2Intr=off  enTzDCBEVT1Intr=off  enTzDCBEVT2Intr=off  ePWMxAforced=No action  ePWMxBforced=No action  DCAEVT1forced=No action  DCBEVT1forced=No action  DCAEVT2forced=No action  DCBEVT2forced=No action  dcah=Trip Zone 1 input (TZ1)  dcal=Trip Zone 1 input (TZ1)  dcbh=Trip Zone 1 input (TZ1)  dcbl=Trip Zone 1 input (TZ1)  dcah_type2=GPTRIP1SEL/(TZ1)  dcal_type2=GPTRIP2SEL/(TZ2)  dcbh_type2=GPTRIP1SEL/(TZ1)  dcbl_type2=GPTRIP2SEL/(TZ2)  gendcaevt1=Event disabled  gendcaevt2=Event disabled  gendcbevt1=Event disabled  gendcbevt2=Event disabled  dcaevt1src=DCAEVT1 with sync  dcaevt2src=DCAEVT2 with sync  dcbevt1src=DCBEVT1 with sync  dcbevt2src=DCBEVT2 with sync  pulsesel=Counter equals to zero (CTR=Zero)  blankinv=off  blankoffset=0  blankwidth=0  evsrcsel=Filtered version of DCAEVT1 (DCAEVT1FILT)  encape=off
      settings: LibrarySourceBlock=c2806xlib/ePWM
  wires:
  Constant6/1 -> Subsystem3/1(kHz)
  Constant7/1 -> Subsystem3/2(%)
  Constant4/1 -> Subsystem1/2(%)
  Subsystem1/1(Out1) -> ePWM3/1
  Constant2/1 -> Subsystem2/1(Hz)
  Subsystem3/2(Out2) -> ePWM2/2
  Subsystem3/1(Out1) -> ePWM2/1
  Constant3/1 -> Subsystem1/1(kHz)
  Constant5/1 -> Subsystem2/2(Duty)
  Subsystem2/1(Out1) -> ePWM1/1
  Subsystem1/2(Out2) -> ePWM3/2
  Subsystem2/2(Out2) -> ePWM1/2
  Constant/1 -> Data Store Write1/1
  Constant1/1 -> Data Store Write2/1
  Unit in Volt/1 -> Gain2/1
  Gain2/1 -> Gain3/1
  Constant8/1 -> Data Store Write4/1
  Constant9/1 -> Data Store Write5/1
  Constant10/1 -> Data Store Write6/1
  Unit in Volt2/1 -> Data Store Write7/1
  Unit in Amp/1 -> Data Store Write3/1
  Debug_OCP/1 -> Data Store Write8/1
  Gain3/1 -> Round/1
  Round/1 -> Data Store Write/1
  Constant12/1 -> Data Store Write9/1
  Debug_OCP1/1 -> Data Store Write10/1
  Constant13/1 -> Data Store Write11/1
  Debug_OCP2/1 -> Data Store Write12/1
  Constant14/1 -> Data Store Write13/1
  Constant11/1 -> Data Store Write14/1
  Constant15/1 -> Data Store Write15/1
  Constant16/1 -> Data Store Write16/1

== system CLA_Sample/Initialize ePWM1 ==

== system CLA_Sample/PWM Update @65KHz ==
  note: This block will update PWM after control calculations.==>
  function : TriggerPort  TriggerType=function-call  VariantControl=(inherit)
  Closed loop PWM generation (Control) : Subsystem  TreatAsAtomicUnit=on
  Fixed Duty update_Phase_A : Subsystem  TreatAsAtomicUnit=on
  Fixed Duty update_Phase_B : Subsystem  TreatAsAtomicUnit=on
  Fixed Duty update_Phase_C : Subsystem  Commented=on  TreatAsAtomicUnit=on
  Function-Call Generator : simulink/Ports & Subsystems/Function-Call Generator  sample_time=-1  numberOfIterations=1  DisallowWideOutput=off
  Function-Call Split : FunctionCallSplit  IconShape=distinctive  NumOutputPorts=4  OutputPortLayout=default
  wires:
  Function-Call Generator/1 -> Function-Call Split/1
  Function-Call Split/1 -> Closed loop PWM generation (Control)/Trigger
  Function-Call Split/2 -> Fixed Duty update_Phase_A/Trigger
  Function-Call Split/3 -> Fixed Duty update_Phase_B/Trigger
  Function-Call Split/4 -> Fixed Duty update_Phase_C/Trigger

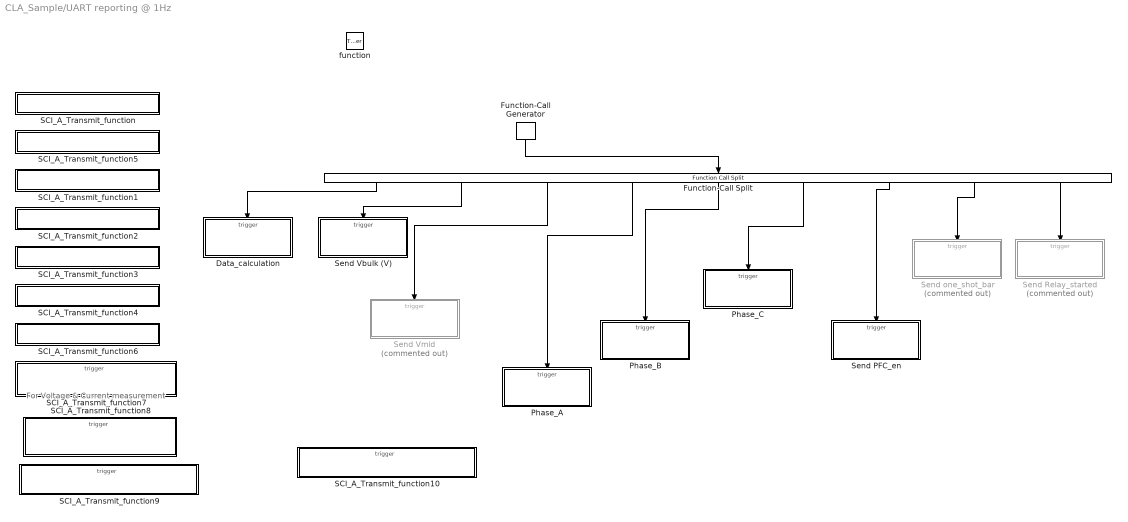
== system CLA_Sample/UART reporting @ 1Hz ==
  note: For Voltage & Current measurement
  function : TriggerPort  TriggerType=function-call  VariantControl=(inherit)
  Data_calculation : Subsystem  TreatAsAtomicUnit=on
  Function-Call Generator : simulink/Ports & Subsystems/Function-Call Generator  sample_time=-1  numberOfIterations=1  DisallowWideOutput=off
  Function-Call Split : FunctionCallSplit  IconShape=distinctive  NumOutputPorts=9  OutputPortLayout=default
  Phase_A : Subsystem  TreatAsAtomicUnit=on
  Phase_B : Subsystem  TreatAsAtomicUnit=on
  Phase_C : Subsystem  TreatAsAtomicUnit=on
  SCI_A_Transmit_function : Subsystem  TreatAsAtomicUnit=on
  SCI_A_Transmit_function1 : Subsystem  TreatAsAtomicUnit=on
  SCI_A_Transmit_function10 : Subsystem  TreatAsAtomicUnit=on
  SCI_A_Transmit_function2 : Subsystem  TreatAsAtomicUnit=on
  SCI_A_Transmit_function3 : Subsystem  TreatAsAtomicUnit=on
  SCI_A_Transmit_function4 : Subsystem  TreatAsAtomicUnit=on
  SCI_A_Transmit_function5 : Subsystem  TreatAsAtomicUnit=on
  SCI_A_Transmit_function6 : Subsystem  TreatAsAtomicUnit=on
  SCI_A_Transmit_function7 : Subsystem  TreatAsAtomicUnit=on
  SCI_A_Transmit_function8 : Subsystem  TreatAsAtomicUnit=on
  SCI_A_Transmit_function9 : Subsystem  TreatAsAtomicUnit=on
  Send PFC_en : Subsystem  TreatAsAtomicUnit=on
  Send Relay_started : Subsystem  Commented=on  TreatAsAtomicUnit=on
  Send Vbulk (V) : Subsystem  TreatAsAtomicUnit=on
  Send Vmid : Subsystem  Commented=on  TreatAsAtomicUnit=on
  Send one_shot_bar : Subsystem  Commented=on  TreatAsAtomicUnit=on
  wires:
  Function-Call Split/2 -> Send Vbulk (V)/Trigger
  Function-Call Generator/1 -> Function-Call Split/1
  Function-Call Split/1 -> Data_calculation/Trigger
  Function-Call Split/3 -> Send Vmid/Trigger
  Function-Call Split/4 -> Phase_A/Trigger
  Function-Call Split/5 -> Phase_B/Trigger
  Function-Call Split/6 -> Phase_C/Trigger
  Function-Call Split/7 -> Send PFC_en/Trigger
  Function-Call Split/8 -> Send one_shot_bar/Trigger
  Function-Call Split/9 -> Send Relay_started/Trigger

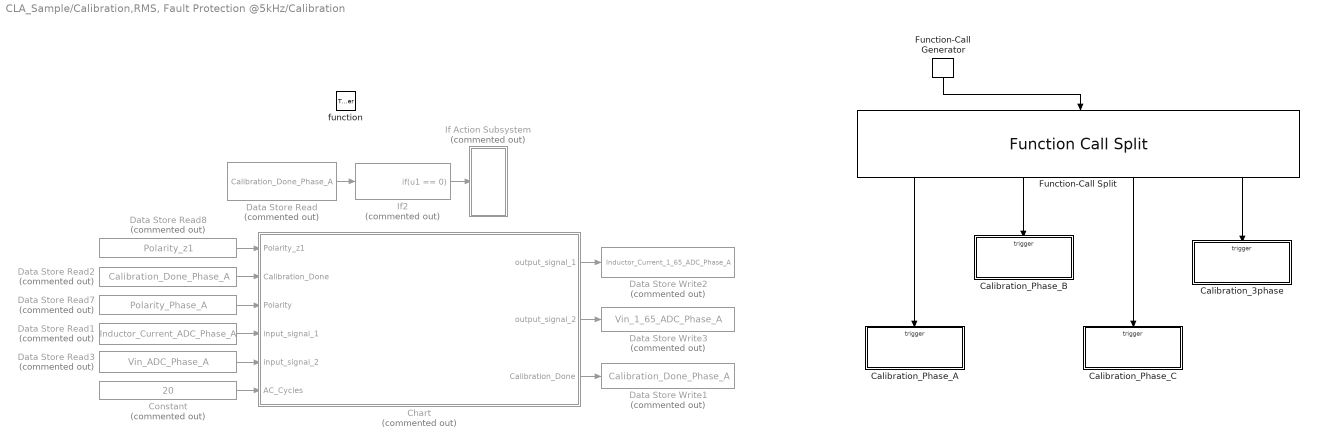
== system CLA_Sample/Calibration,RMS, Fault Protection @5kHz/Calibration ==
  function : TriggerPort  TriggerType=function-call  VariantControl=(inherit)
  Calibration_3phase : Subsystem  TreatAsAtomicUnit=on
  Calibration_Phase_A : Subsystem  TreatAsAtomicUnit=on
  Calibration_Phase_B : Subsystem  TreatAsAtomicUnit=on
  Calibration_Phase_C : Subsystem  TreatAsAtomicUnit=on
  Chart : Stateflow chart  Commented=on  TreatAsAtomicUnit=on
  Constant : Constant  Commented=on  Value=20
  Data Store Read : DataStoreRead  Commented=on  DataStoreName=Calibration_Done_Phase_A  IndexOptions=Index vector (dialog)  Indices=1  OutputSizes=1
  Data Store Read1 : DataStoreRead  Commented=on  DataStoreName=Inductor_Current_ADC_Phase_A  IndexOptions=Index vector (dialog)  Indices=1  OutputSizes=1
  Data Store Read2 : DataStoreRead  Commented=on  DataStoreName=Calibration_Done_Phase_A  IndexOptions=Index vector (dialog)  Indices=1  OutputSizes=1
  Data Store Read3 : DataStoreRead  Commented=on  DataStoreName=Vin_ADC_Phase_A  IndexOptions=Index vector (dialog)  Indices=1  OutputSizes=1
  Data Store Read7 : DataStoreRead  Commented=on  DataStoreName=Polarity_Phase_A  IndexOptions=Index vector (dialog)  Indices=1  OutputSizes=1
  Data Store Read8 : DataStoreRead  Commented=on  DataStoreName=Polarity_z1  IndexOptions=Index vector (dialog)  Indices=1  OutputSizes=1
  Data Store Write1 : DataStoreWrite  Commented=on  DataStoreName=Calibration_Done_Phase_A  IndexOptions=Index vector (dialog)  Indices=1  OutputSizes=1
  Data Store Write2 : DataStoreWrite  Commented=on  DataStoreName=Inductor_Current_1_65_ADC_Phase_A  IndexOptions=Index vector (dialog)  Indices=1  OutputSizes=1
  Data Store Write3 : DataStoreWrite  Commented=on  DataStoreName=Vin_1_65_ADC_Phase_A  IndexOptions=Index vector (dialog)  Indices=1  OutputSizes=1
  Function-Call Generator : simulink/Ports & Subsystems/Function-Call Generator  sample_time=-1  numberOfIterations=1  DisallowWideOutput=off
  Function-Call Split : FunctionCallSplit  IconShape=distinctive  NumOutputPorts=4  OutputPortLayout=default
  If Action Subsystem : Subsystem  Commented=on  TreatAsAtomicUnit=on
  If2 : If  Commented=on  IfExpression=u1 == 0  ShowElse=off
  wires:
  If2/1 -> If Action Subsystem/Action
  Data Store Read/1 -> If2/1
  Data Store Read1/1 -> Chart/4(input_signal_1)
  Data Store Read2/1 -> Chart/2("Calibration_Done ")
  Data Store Read3/1 -> Chart/5(input_signal_2)
  Constant/1 -> Chart/6(AC_Cycles)
  Chart/1(output_signal_1) -> Data Store Write2/1
  Chart/3(Calibration_Done) -> Data Store Write1/1
  Chart/2(output_signal_2) -> Data Store Write3/1
  Data Store Read7/1 -> Chart/3(Polarity)
  Data Store Read8/1 -> Chart/1(Polarity_z1)
  Function-Call Generator/1 -> Function-Call Split/1
  Function-Call Split/2 -> Calibration_Phase_B/Trigger
  Function-Call Split/1 -> Calibration_Phase_A/Trigger
  Function-Call Split/3 -> Calibration_Phase_C/Trigger
  Function-Call Split/4 -> Calibration_3phase/Trigger

== system CLA_Sample/Calibration,RMS, Fault Protection @5kHz/Fault checking ==
  function : TriggerPort  TriggerType=function-call  VariantControl=(inherit)
  Data Store Read4 : DataStoreRead  DataStoreName=Calibration_Done  IndexOptions=Index vector (dialog)  Indices=1  OutputSizes=1
  If : If  IfExpression=u1 ==1  ShowElse=off
  If Action Subsystem : Subsystem  TreatAsAtomicUnit=on
  wires:
  If/1 -> If Action Subsystem/Action
  Data Store Read4/1 -> If/1

== system CLA_Sample/Calibration,RMS, Fault Protection @5kHz/Polarity & Near Zero check ==
  function : TriggerPort  TriggerType=function-call  VariantControl=(inherit)
  Function-Call Generator : simulink/Ports & Subsystems/Function-Call Generator  sample_time=-1  numberOfIterations=1  DisallowWideOutput=off
  Function-Call Split : FunctionCallSplit  IconShape=distinctive  NumOutputPorts=3  OutputPortLayout=default
  Polarity_Near_zero_Phase_A : Subsystem  TreatAsAtomicUnit=on
  Polarity_Near_zero_Phase_B : Subsystem  TreatAsAtomicUnit=on
  Polarity_Near_zero_Phase_C : Subsystem  TreatAsAtomicUnit=on
  wires:
  Function-Call Generator/1 -> Function-Call Split/1
  Function-Call Split/1 -> Polarity_Near_zero_Phase_A/Trigger
  Function-Call Split/2 -> Polarity_Near_zero_Phase_B/Trigger
  Function-Call Split/3 -> Polarity_Near_zero_Phase_C/Trigger
